simulink model "cordic_sysgen_cosim"  (R2017a)
settings: Solver=VariableStepAuto  StartTime=0.0  StopTime=14801  RelTol=1e-3
undefined symbols (not defined in the file or in its folder): A, N
libraries: xbsIndex_r4 x20, JTAGRuntimeCosim_r4 x1
settings Model: Creator=jhell  LastModifiedBy=jlh24

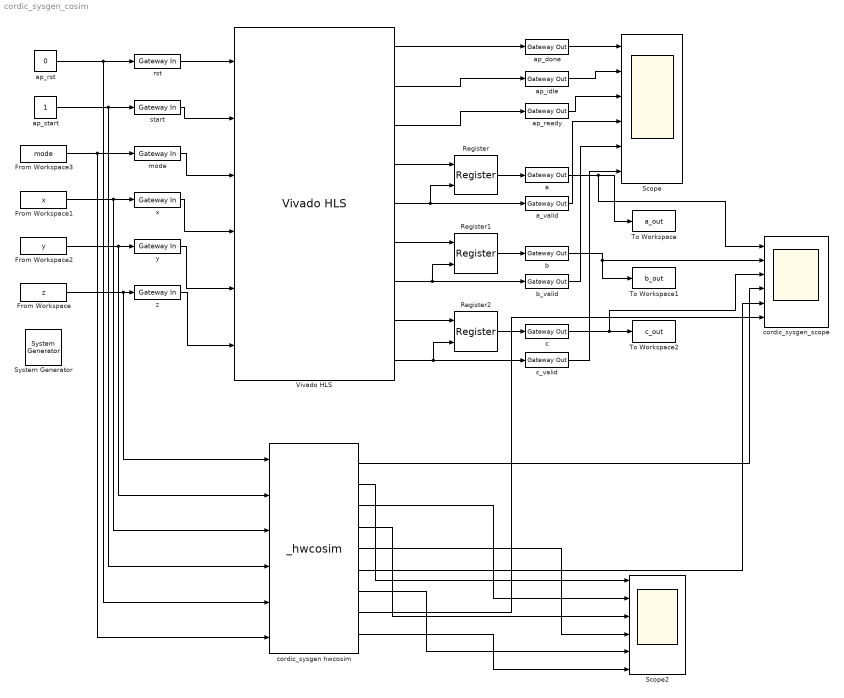
== system cordic_sysgen_cosim ==
  " System Generator" : xbsIndex_r4/ System Generator  Tag=genX  xilinxfamily=zynq  part=xc7z020  speed=-1  package=clg484  synthesis_tool=Vivado  clock_wrapper=Clock Enables  directory=./netlist  proj_type=Vivado  Synth_file=Vivado Synthesis Defaults  Impl_file=Vivado Implementation Defaults  testbench=off  simulink_period=1  sysclk_period=10  dcm_input_clock_period=10  incr_netlist=off  trim_vbits=Everywhere in SubSystem  dbl_ovrd=According to Block Masks  core_generation=According to Block Masks  run_coregen=off  deprecated_control=off  eval_field=0  block_type=sysgen
  From Workspace : FromWorkspace  VariableName=z  SampleTime=0  Interpolate=off  OutputAfterFinalValue=Setting to zero
  From Workspace1 : FromWorkspace  VariableName=x  SampleTime=0  Interpolate=off  OutputAfterFinalValue=Setting to zero
  From Workspace2 : FromWorkspace  VariableName=y  SampleTime=0  Interpolate=off  OutputAfterFinalValue=Setting to zero
  From Workspace3 : FromWorkspace  VariableName=mode  SampleTime=0  Interpolate=off  OutputAfterFinalValue=Setting to zero
  Register : xbsIndex_r4/Register  init=0  rst=off  en=on  dbl_ovrd=off  block_type=register
  Register1 : xbsIndex_r4/Register  init=0  rst=off  en=on  dbl_ovrd=off  block_type=register
  Register2 : xbsIndex_r4/Register  init=0  rst=off  en=on  dbl_ovrd=off  block_type=register
  Scope : Scope  NumInputPorts=6
  Scope2 : Scope  NumInputPorts=6
  To Workspace : ToWorkspace  VariableName=a_out  SampleTime=-1
  To Workspace1 : ToWorkspace  VariableName=b_out  SampleTime=-1
  To Workspace2 : ToWorkspace  VariableName=c_out  SampleTime=-1
  Vivado HLS : xbsIndex_r4/Vivado HLS  anytable='C:/ELEC522/hellar/Project_4/cordic_revised/cordic_revised/solution1'  fast_sim=off  display_datatype=on  rate_propagation_method=Simulink system period  model_file_path=''  latency=1  block_type=hls
      settings: infoedit=This block allows including C,C++ and SystemC source files in System Generator for DSP designs.
  a : xbsIndex_r4/Gateway Out  inherit_from_input=off  hdl_port=on  rows=1  columns=1  UseAsDAC=off  DACChannel='1'  interface=None  automatic_assignment=on  address_offset=hex2dec('00')  intf_name=''  intf_description=''  timing_constraint=None  locs_specified=off  LOCs={}  io_standard={}  block_type=gatewayout
  a_valid : xbsIndex_r4/Gateway Out  inherit_from_input=off  hdl_port=on  rows=1  columns=1  UseAsDAC=off  DACChannel='1'  interface=None  automatic_assignment=on  address_offset=hex2dec('00')  intf_name=''  intf_description=''  timing_constraint=None  locs_specified=off  LOCs={}  io_standard={}  block_type=gatewayout
  ap_done : xbsIndex_r4/Gateway Out  inherit_from_input=off  hdl_port=on  rows=1  columns=1  UseAsDAC=off  DACChannel='1'  interface=None  automatic_assignment=on  address_offset=hex2dec('00')  intf_name=''  intf_description=''  timing_constraint=None  locs_specified=off  LOCs={}  io_standard={}  block_type=gatewayout
  ap_idle : xbsIndex_r4/Gateway Out  inherit_from_input=off  hdl_port=on  rows=1  columns=1  UseAsDAC=off  DACChannel='1'  interface=None  automatic_assignment=on  address_offset=hex2dec('00')  intf_name=''  intf_description=''  timing_constraint=None  locs_specified=off  LOCs={}  io_standard={}  block_type=gatewayout
  ap_ready : xbsIndex_r4/Gateway Out  inherit_from_input=off  hdl_port=on  rows=1  columns=1  UseAsDAC=off  DACChannel='1'  interface=None  automatic_assignment=on  address_offset=hex2dec('00')  intf_name=''  intf_description=''  timing_constraint=None  locs_specified=off  LOCs={}  io_standard={}  block_type=gatewayout
  ap_rst : Constant  Value=0
  ap_start : Constant
  b : xbsIndex_r4/Gateway Out  inherit_from_input=off  hdl_port=on  rows=1  columns=1  UseAsDAC=off  DACChannel='1'  interface=None  automatic_assignment=on  address_offset=hex2dec('00')  intf_name=''  intf_description=''  timing_constraint=None  locs_specified=off  LOCs={}  io_standard={}  block_type=gatewayout
  b_valid : xbsIndex_r4/Gateway Out  inherit_from_input=off  hdl_port=on  rows=1  columns=1  UseAsDAC=off  DACChannel='1'  interface=None  automatic_assignment=on  address_offset=hex2dec('00')  intf_name=''  intf_description=''  timing_constraint=None  locs_specified=off  LOCs={}  io_standard={}  block_type=gatewayout
  c : xbsIndex_r4/Gateway Out  inherit_from_input=off  hdl_port=on  rows=1  columns=1  UseAsDAC=off  DACChannel='1'  interface=None  automatic_assignment=on  address_offset=hex2dec('00')  intf_name=''  intf_description=''  timing_constraint=None  locs_specified=off  LOCs={}  io_standard={}  block_type=gatewayout
  c_valid : xbsIndex_r4/Gateway Out  inherit_from_input=off  hdl_port=on  rows=1  columns=1  UseAsDAC=off  DACChannel='1'  interface=None  automatic_assignment=on  address_offset=hex2dec('00')  intf_name=''  intf_description=''  timing_constraint=None  locs_specified=off  LOCs={}  io_standard={}  block_type=gatewayout
  cordic_sysgen hwcosim : JTAGRuntimeCosim_r4/_hwcosim  clkSrc=Single Stepped  hasCombinationalPath=on  bitfileName=C:\ELEC522\hellar\Project_4\netlist\cordic_sysgen.bit  skipConfig=off  dispPartInfo=off  useZynqReconfigScript=on  cable=Auto Detect  speed=N/A  cablePort=N/A  cableLocation=Local  shareCable=off  design_xtable=|  engineDll=JTAGCosimEngine.dll  cableWaitTime=10  bscanPos=-1  IRLengths=[]  useWaitBox=1  hasBufgmux=on  Scheme=Cosim  useCmdProc=1  hasProc=0  useImpact=0  printLogFile=0  userChain=2  block_type=jtagcosim
      | {
      |     'clkWrapper' => 'cordic_sysgen',
      |     'burstMode' => false,
      |     'burstFifoDepth' => '1024',
      |     'shared_memories' => {},
      |     'clocksGcd' => 1,
      |     'device' => {
      |       'family' => 'zynq',
      |       'part' => 'xc7z020',
      |       'package' => 'clg484',
      |       'speed' => '-1',
      |     },
      |     'ports' => {
      |       'z' => {
      |         'direction' => 'in',
      |         'width' => 16,
      |         'name' => 'z',
      |         'period' => 1,
      |         'icon_text' => 'z',
      |         'type' => 'Fix_16_13',
      |         'arithmetic_type' => 'xlSigned',
      |         'dat_file' => 'cordic_sysgen_z.dat',
      |         'bin_pt' => 13,
      |         'addr_offset' => 0,
      |         'bd_port_index' => 0,
      |       },
      |       'y' => {
      |         'direction' => 'in',
      |         'width' => 16,
      |         'name' => 'y',
      |         'period' => 1,
      |         'icon_text' => 'y',
      |         'type' => 'Fix_16_13',
      |         'arithmetic_type' => 'xlSigned',
      |         'dat_file' => 'cordic_sysgen_y.dat',
      |         'bin_pt' => 13,
      |         'addr_offset' => 4,
      |         'bd_port_index' => 1,
      |       },
      |       'x' => {
      |         'direction' => 'in',
      |         'width' => 16,
      |         'name' => 'x',
      |         'period' => 1,
      |         'icon_text' => 'x',
      |         'type' => 'Fix_16_13',
      |         'arithmetic_type' => 'xlSigned',
      |         'dat_file' => 'cordic_sysgen_x.dat',
      |         'bin_pt' => 13,
      |         'addr_offset' => 8,
      |         'bd_port_index' => 2,
      |       },
      |       'start' => {
      |         'direction' => 'in',
      |         'width' => 1,
      |         'name' => 'start',
      |         'period' => 1,
      |         'icon_text' => 'start',
      |         'type' => 'Bool',
      |         'arithmetic_type' => 'xlUnsigned',
      |         'dat_file' => 'cordic_sysgen_start.dat',
      |         'bin_pt' => 0,
      |         'addr_offset' => 12,
      |         'bd_port_index' => 3,
      |       },
      |       'rst' => {
      |         'direction' => 'in',
      |         'width' => 1,
      |         'name' => 'rst',
      |         'period' => 1,
      |         'icon_text' => 'rst',
      |         'type' => 'Bool',
      |         'arithmetic_type' => 'xlUnsigned',
      |         'dat_file' => 'cordic_sysgen_rst.dat',
      |         'bin_pt' => 0,
      |         'addr_offset' => 16,
      |         'bd_port_index' => 4,
      |       },
      |       'mode' => {
      |         'direction' => 'in',
      |         'width' => 1,
      |         'name' => 'mode',
      |         'period' => 1,
      |         'icon_text' => 'mode',
      |         'type' => 'Bool',
      |         'arithmetic_type' => 'xlUnsigned',
      |         'dat_file' => 'cordic_sysgen_mode.dat',
      |         'bin_pt' => 0,
      |         'addr_offset' => 20,
      |         'bd_port_index' => 5,
      |       },
      |       'a' => {
      |         'direction' => 'out',
      |         'width' => 16,
      |         'name' => 'a',
      |         'period' => 1,
      |         'icon_text' => 'a',
      |         'type' => 'Fix_16_13',
      |         'arithmetic_type' => 'xlSigned',
      |         'dat_file' => 'cordic_sysgen_a.dat',
      |         'bin_pt' => 13,
      |         'addr_offset' => 24,
      |         'bd_port_index' => 0,
      |       },
      |       'a_valid' => {
      |         'direction' => 'out',
      |         'width' => 1,
      |         'name' => 'a_valid',
      |         'period' => 1,
      |         'icon_text' => 'a_valid',
      |         'type' => 'Bool',
      |         'arithmetic_type' => 'xlUnsigned',
      |         'dat_file' => 'cordic_sysgen_a_valid.dat',
      |         'bin_pt' => 0,
      |         'addr_offset' => 28,
      |         'bd_port_index' => 1,
      |       },
      |       'ap_done' => {
      |         'direction' => 'out',
      |         'width' => 1,
      |         'name' => 'ap_done',
      |         'period' => 1,
      |         'icon_text' => 'ap_done',
      |         'type' => 'Bool',
      |         'arithmetic_type' => 'xlUnsigned',
      |         'dat_file' => 'cordic_sysgen_ap_done.dat',
      |         'bin_pt' => 0,
      |         'addr_offset' => 32,
      |         'bd_port_index' => 2,
      |       },
      |       'ap_idle' => {
      |         'direction' => 'out',
      |         'width' => 1,
      |         'name' => 'ap_idle',
      |         'period' => 1,
      |         'icon_text' => 'ap_idle',
      |         'type' => 'Bool',
      |         'arithmetic_type' => 'xlUnsigned',
      |         'dat_file' => 'cordic_sysgen_ap_idle.dat',
      |         'bin_pt' => 0,
      |         'addr_offset' => 36,
      |         'bd_port_index' => 3,
      |       },
      |       'ap_ready' => {
      |         'direction' => 'out',
      |         'width' => 1,
      |         'name' => 'ap_ready',
      |         'period' => 1,
      |         'icon_text' => 'ap_ready',
      |         'type' => 'Bool',
      |         'arithmetic_type' => 'xlUnsigned',
      |         'dat_file' => 'cordic_sysgen_ap_ready.dat',
      |         'bin_pt' => 0,
      |         'addr_offset' => 40,
      |         'bd_port_index' => 4,
      |       },
      |       'b' => {
      |         'direction' => 'out',
      |         'width' => 16,
      |         'name' => 'b',
      |         'period' => 1,
      |         'icon_text' => 'b',
      |         'type' => 'Fix_16_13',
      |         'arithmetic_type' => 'xlSigned',
      |         'dat_file' => 'cordic_sysgen_b.dat',
      |         'bin_pt' => 13,
      |         'addr_offset' => 44,
      |         'bd_port_index' => 5,
      |       },
      |       'b_valid' => {
      |         'direction' => 'out',
      |         'width' => 1,
      |         'name' => 'b_valid',
      |         'period' => 1,
      |         'icon_text' => 'b_valid',
      |         'type' => 'Bool',
      |         'arithmetic_type' => 'xlUnsigned',
      |         'dat_file' => 'cordic_sysgen_b_valid.dat',
      |         'bin_pt' => 0,
      |         'addr_offset' => 48,
      |         'bd_port_index' => 6,
      |       },
      |       'c' => {
      |         'direction' => 'out',
      |         'width' => 16,
      |         'name' => 'c',
      |         'period' => 1,
      |         'icon_text' => 'c',
      |         'type' => 'Fix_16_13',
      |         'arithmetic_type' => 'xlSigned',
      |         'dat_file' => 'cordic_sysgen_c.dat',
      |         'bin_pt' => 13,
      |         'addr_offset' => 52,
      |         'bd_port_index' => 7,
      |       },
      |       'c_valid' => {
      |         'direction' => 'out',
      |         'width' => 1,
      |         'name' => 'c_valid',
      |         'period' => 1,
      |         'icon_text' => 'c_valid',
      |         'type' => 'Bool',
      |         'arithmetic_type' => 'xlUnsigned',
      |         'dat_file' => 'cordic_sysgen_c_valid.dat',
      |         'bin_pt' => 0,
      |         'addr_offset' => 56,
      |         'bd_port_index' => 8,
      |       },
      |     },
      |   }
  cordic_sysgen_scope : Scope  NumInputPorts=6
  mode : xbsIndex_r4/Gateway In  gui_display_data_type=Boolean  arith_type=Boolean  n_bits=16  bin_pt=14  preci_type=Single  exp_width=8  frac_width=24  rows=1  columns=1  quantization="Round  (unbiased: +/- Inf)"  overflow=Saturate  period=1  UseAsADC=off  ADCChannel='1'  interface=None  automatic_assignment=on  address_offset=hex2dec('00')  intf_name=''  intf_description=''  default_value=0  timing_constraint=None  locs_specified=off  LOCs={}  io_standard={}  inherit_from_input=off  hdl_port=on  dbl_ovrd=off  block_type=gatewayin
  rst : xbsIndex_r4/Gateway In  gui_display_data_type=Boolean  arith_type=Boolean  n_bits=16  bin_pt=14  preci_type=Single  exp_width=8  frac_width=24  rows=1  columns=1  quantization="Round  (unbiased: +/- Inf)"  overflow=Saturate  period=1  UseAsADC=off  ADCChannel='1'  interface=None  automatic_assignment=on  address_offset=hex2dec('00')  intf_name=''  intf_description=''  default_value=0  timing_constraint=None  locs_specified=off  LOCs={}  io_standard={}  inherit_from_input=off  hdl_port=on  dbl_ovrd=off  block_type=gatewayin
  start : xbsIndex_r4/Gateway In  gui_display_data_type=Boolean  arith_type=Boolean  n_bits=16  bin_pt=14  preci_type=Single  exp_width=8  frac_width=24  rows=1  columns=1  quantization="Round  (unbiased: +/- Inf)"  overflow=Saturate  period=1  UseAsADC=off  ADCChannel='1'  interface=None  automatic_assignment=on  address_offset=hex2dec('00')  intf_name=''  intf_description=''  default_value=0  timing_constraint=None  locs_specified=off  LOCs={}  io_standard={}  inherit_from_input=off  hdl_port=on  dbl_ovrd=off  block_type=gatewayin
  x : xbsIndex_r4/Gateway In  gui_display_data_type=Fixed-point  arith_type="Signed  (2's comp)"  n_bits=16  bin_pt=13  preci_type=Single  exp_width=8  frac_width=24  rows=1  columns=1  quantization="Round  (unbiased: +/- Inf)"  overflow=Saturate  period=1  UseAsADC=off  ADCChannel='1'  interface=None  automatic_assignment=on  address_offset=hex2dec('00')  intf_name=''  intf_description=''  default_value=0  timing_constraint=None  locs_specified=off  LOCs={}  io_standard={}  inherit_from_input=off  hdl_port=on  dbl_ovrd=off  block_type=gatewayin
  y : xbsIndex_r4/Gateway In  gui_display_data_type=Fixed-point  arith_type="Signed  (2's comp)"  n_bits=16  bin_pt=13  preci_type=Single  exp_width=8  frac_width=24  rows=1  columns=1  quantization="Round  (unbiased: +/- Inf)"  overflow=Saturate  period=1  UseAsADC=off  ADCChannel='1'  interface=None  automatic_assignment=on  address_offset=hex2dec('00')  intf_name=''  intf_description=''  default_value=0  timing_constraint=None  locs_specified=off  LOCs={}  io_standard={}  inherit_from_input=off  hdl_port=on  dbl_ovrd=off  block_type=gatewayin
  z : xbsIndex_r4/Gateway In  gui_display_data_type=Fixed-point  arith_type="Signed  (2's comp)"  n_bits=16  bin_pt=13  preci_type=Single  exp_width=8  frac_width=24  rows=1  columns=1  quantization="Round  (unbiased: +/- Inf)"  overflow=Saturate  period=1  UseAsADC=off  ADCChannel='1'  interface=None  automatic_assignment=on  address_offset=hex2dec('00')  intf_name=''  intf_description=''  default_value=0  timing_constraint=None  locs_specified=off  LOCs={}  io_standard={}  inherit_from_input=off  hdl_port=on  dbl_ovrd=off  block_type=gatewayin
  wires:
  ap_rst/1 -> cordic_sysgen hwcosim/5, rst/1
  rst/1 -> Vivado HLS/1
  ap_start/1 -> cordic_sysgen hwcosim/4, start/1
  start/1 -> Vivado HLS/2
  From Workspace3/1 -> cordic_sysgen hwcosim/6, mode/1
  mode/1 -> Vivado HLS/3
  From Workspace1/1 -> cordic_sysgen hwcosim/3, x/1
  x/1 -> Vivado HLS/4
  From Workspace2/1 -> cordic_sysgen hwcosim/2, y/1
  From Workspace/1 -> cordic_sysgen hwcosim/1, z/1
  z/1 -> Vivado HLS/6
  Vivado HLS/1 -> ap_done/1
  ap_done/1 -> Scope/1
  Vivado HLS/5 -> Register/2, a_valid/1
  Vivado HLS/7 -> Register1/2, b_valid/1
  Vivado HLS/9 -> Register2/2, c_valid/1
  Vivado HLS/2 -> ap_idle/1
  Vivado HLS/3 -> ap_ready/1
  ap_idle/1 -> Scope/2
  ap_ready/1 -> Scope/3
  a_valid/1 -> Scope/4
  b_valid/1 -> Scope/5
  c_valid/1 -> Scope/6
  a/1 -> cordic_sysgen_scope/1, To Workspace/1
  c/1 -> cordic_sysgen_scope/3, To Workspace2/1
  Vivado HLS/4 -> Register/1
  Register/1 -> a/1
  Vivado HLS/6 -> Register1/1
  Register1/1 -> b/1
  Vivado HLS/8 -> Register2/1
  Register2/1 -> c/1
  y/1 -> Vivado HLS/5
  b/1 -> cordic_sysgen_scope/2, To Workspace1/1
  cordic_sysgen hwcosim/9 -> Scope2/6
  cordic_sysgen hwcosim/7 -> Scope2/5
  cordic_sysgen hwcosim/5 -> Scope2/4
  cordic_sysgen hwcosim/3 -> Scope2/2
  cordic_sysgen hwcosim/4 -> Scope2/3
  cordic_sysgen hwcosim/2 -> Scope2/1
  cordic_sysgen hwcosim/1 -> cordic_sysgen_scope/4
  cordic_sysgen hwcosim/6 -> cordic_sysgen_scope/5
  cordic_sysgen hwcosim/8 -> cordic_sysgen_scope/6
